simulink model "control_system"  (R2022a)
settings: Solver=VariableStepAuto  StartTime=0.0  StopTime=10.0  RelTol=1e-3
values from neighbouring files (symbols this model uses):
  a = 0.25    [control_system_settings.m]
  b = 2    [control_system_settings.m]
  k = 1.2    [control_system_settings.m]
settings Model: Creator=Home computer  LastModifiedBy=Home computer

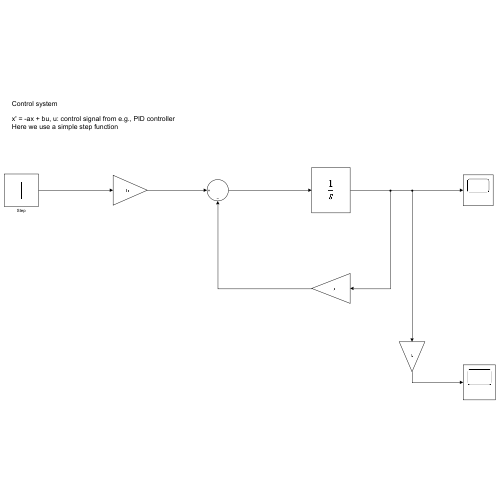
[thumbnail: Simulink's stored preview of the top-level diagram]
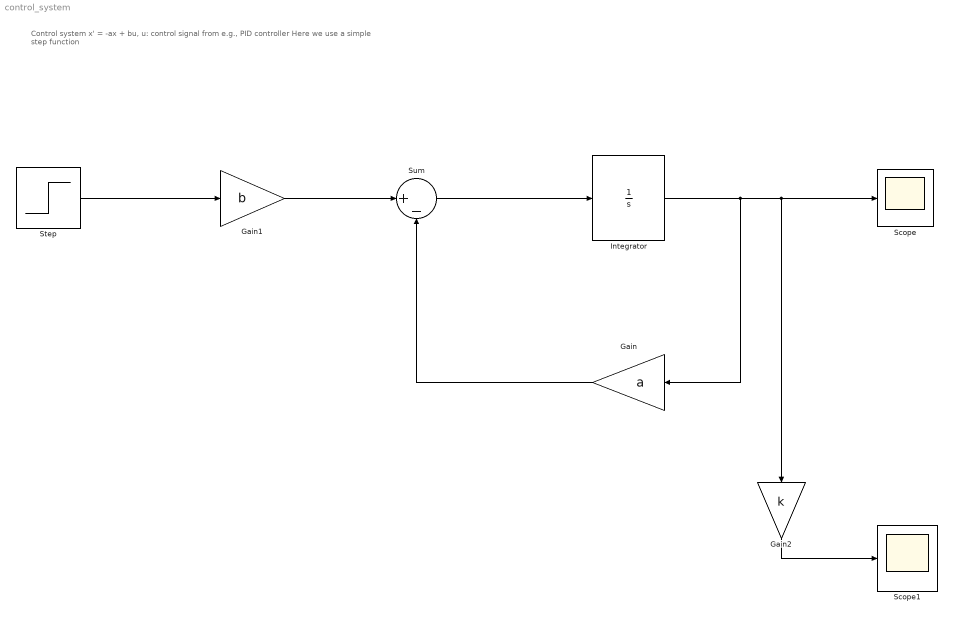
== system control_system ==
  note: Control system
      |
      | x' = -ax + bu, u: control signal from e.g., PID controller
      | Here we use a simple step function
  Gain : Gain  Gain=a
  Gain1 : Gain  Gain=b
  Gain2 : Gain  Gain=k
  Integrator : Integrator
  Scope : Scope
  Scope1 : Scope
  Step : Step  SampleTime=0
  Sum : Sum  Inputs=|+-
  wires:
  Integrator/1 -> Scope/1, Gain2/1, Gain/1
  Gain/1 -> Sum/2
  Sum/1 -> Integrator/1
  Gain1/1 -> Sum/1
  Step/1 -> Gain1/1
  Gain2/1 -> Scope1/1
